simulink model "chap3_7sim"  (Simulink 5.0)
settings: Solver=ode45  StartTime=0.0  StopTime=10  FixedStep=0.001  RelTol=1e-3
settings Model: LastModifiedBy=Administrator  ExtModeTrigMode=oneshot  ExtModeArmWhenConnect=off  LimitDataPoints=off  BooleanDataType=off

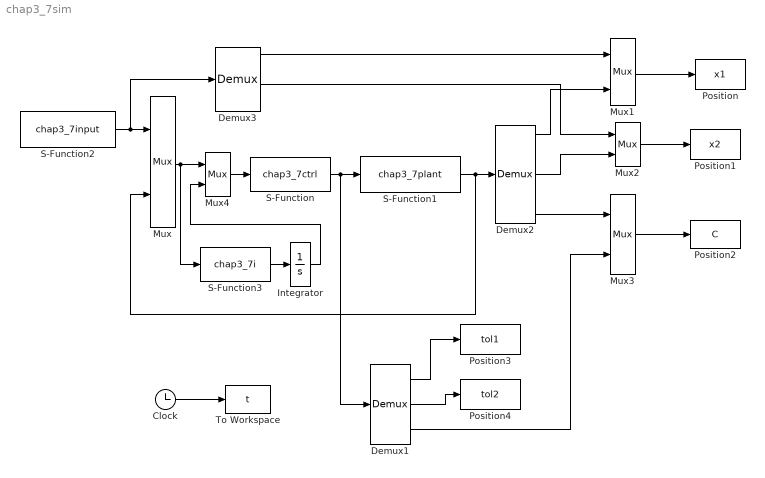
== system chap3_7sim ==
  Clock : Clock
      settings: Decimation=10
  Demux1 : Demux  Outputs=3
  Demux2 : Demux  Outputs=5
  Demux3 : Demux  Outputs=6
  Integrator : Integrator
  Mux{,1..4} (5 alike) : Mux  Inputs=2
  Position : ToWorkspace  VariableName=x1  SampleTime=-1  SaveFormat=Array
  Position1 : ToWorkspace  VariableName=x2  SampleTime=-1  SaveFormat=Array
  Position2 : ToWorkspace  VariableName=C  SampleTime=-1  SaveFormat=Array
  Position3 : ToWorkspace  VariableName=tol1  SampleTime=-1  SaveFormat=Array
  Position4 : ToWorkspace  VariableName=tol2  SampleTime=-1  SaveFormat=Array
  S-Function : S-Function  FunctionName=chap3_7ctrl
  S-Function1 : S-Function  FunctionName=chap3_7plant
  S-Function2 : S-Function  FunctionName=chap3_7input
  S-Function3 : S-Function  FunctionName=chap3_7i
  To Workspace : ToWorkspace  VariableName=t  SampleTime=-1  SaveFormat=Array
  wires:
  Mux/1 -> S-Function3/1, Mux4/1
  Demux2/1 -> Mux1/2
  S-Function1/1 -> Demux2/1, Mux/2
  S-Function2/1 -> Demux3/1, Mux/1
  Demux1/1 -> Position3/1
  Demux1/2 -> Position4/1
  Demux3/1 -> Mux1/1
  Mux1/1 -> Position/1
  Mux2/1 -> Position1/1
  S-Function/1 -> S-Function1/1, Demux1/1
  Mux3/1 -> Position2/1
  Demux1/3 -> Mux3/2
  Demux2/5 -> Mux3/1
  Mux4/1 -> S-Function/1
  S-Function3/1 -> Integrator/1
  Integrator/1 -> Mux4/2
  Demux3/4 -> Mux2/1
  Demux2/3 -> Mux2/2
  Clock/1 -> To Workspace/1
